simulink library "inp"  (R2021b)
settings: Solver=VariableStepAuto  StartTime=0.0  StopTime=10.0  RelTol=1e-3
undefined symbols (not defined in the file): C_TASK_5MS_S, FALSE, KINP_AcoreReadyToSlp_flg_ovrdflg, KINP_AcoreReadyToSlp_flg_ovrdval, KINP_AllowMovThd_OTA_enum_ovrdflg, KINP_AllowMovThd_OTA_enum_ovrdval, KINP_APSAngleTarget_Deg_ovrdflg, KINP_APSAngleTarget_Deg_ovrdval, KINP_APSDecReq_mps2_ovrdflg, KINP_APSDecReq_mps2_ovrdval, KINP_APSDecReqA_flg_ovrdflg, KINP_APSDecReqA_flg_ovrdval, KINP_APSDFLL_cm_ovrdflg, KINP_APSDFLL_cm_ovrdval, KINP_APSDFLR_cm_ovrdflg, KINP_APSDFLR_cm_ovrdval, KINP_APSDRLL_cm_ovrdflg, KINP_APSDRLL_cm_ovrdval, KINP_APSDRLR_cm_ovrdflg, KINP_APSDRLR_cm_ovrdval, KINP_APSExitCondition_enum_ovrdflg, KINP_APSExitCondition_enum_ovrdval, KINP_APSHWVer_enum_ovrdflg, KINP_APSHWVer_enum_ovrdval, KINP_APSProgressPCT_pct_ovrdflg, KINP_APSProgressPCT_pct_ovrdval, KINP_APSReq_enum_ovrdflg, KINP_APSReq_enum_ovrdval, KINP_APSRQDisplay_enum_ovrdflg, KINP_APSRQDisplay_enum_ovrdval, KINP_APSRqEPASCtrl_flg_ovrdflg, KINP_APSRqEPASCtrl_flg_ovrdval, KINP_APSShiftPosnReq_enum_ovrdval, KINP_APSShiftPosnReq_enum_ovrflg, KINP_APSSpeedCMD_kph_ovrdval, KINP_APSSpeedCMD_kph_ovrflg, KINP_APSStaSystem_enum_ovrdflg, KINP_APSStaSystem_enum_ovrdval, KINP_APSSWVer_enum_ovrdflg, KINP_APSSWVer_enum_ovrdval, KINP_APSVMCReqA_flg_ovrdval, KINP_APSVMCReqA_flg_ovrflg, KINP_APSVRqEPASCtrl_flg_ovrdflg, KINP_APSVRqEPASCtrl_flg_ovrdval, KINP_AuxBattVolmV_mV_ovrdflg, KINP_AuxBattVolmV_mV_ovrdval, KINP_CAASSta_enum_ovrdflg, KINP_CAASSta_enum_ovrdval, KINP_CAASVMCReqA_flg_ovrdval, KINP_CAASVMCReqA_flg_ovrflg, KINP_Chime_enum_ovrdflg, KINP_Chime_enum_ovrdval, KINP_ClearDTCcmd_flg_ovrdflg, KINP_ClearDTCcmd_flg_ovrdval, KINP_EvccAplusPwrUpReq_flg_ovrdflg, KINP_EvccAplusPwrUpReq_flg_ovrdval, KINP_LFID_raw_ovrdval, KINP_LFID_raw_ovrflg, KINP_LRID_raw_ovrdval, KINP_MemOffsetAccX_raw16_ovrdflg ... (+118)
libraries: FVT_lib x595, hcu_lib x1
(part 13 of 27)

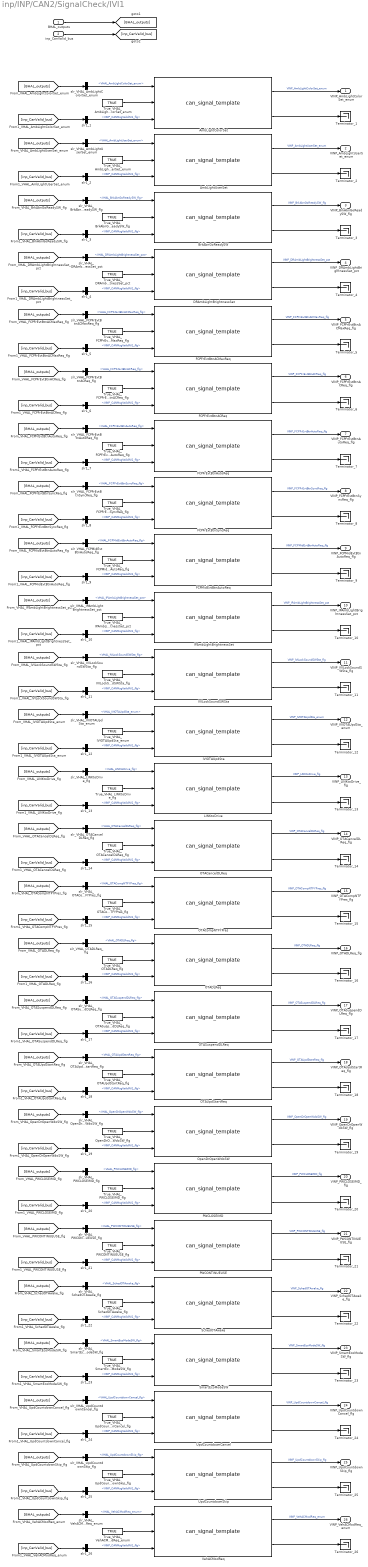
== system inp/INP/CAN2/SignalCheck/IVI1 ==
  BHAL_outputs : Inport
  inp_CanValid_bus : Inport  Port=2
  AmbLightColorSet : FVT_lib/inp/can_signal_template  SystemSampleTime=-1  VariantActivationTime=update diagram  Latency=0  AutoFrameSizeCalculation=off
      link override defval: Value=KINP_AmbLightColorSet_enum_defval
      link override fftdec: Value=KINP_AmbLightColorSet_enum_fftdec
      link override fftinc: Value=KINP_AmbLightColorSet_enum_fftinc
      link override fftlim: Value=KINP_AmbLightColorSet_enum_fftlim
      link override invalid: Value=KINP_AmbLightColorSet_enum_invalid
      link override ovrdflg: Value=KINP_AmbLightColorSet_enum_ovrdflg
      link override ovrdval: Value=KINP_AmbLightColorSet_enum_ovrdval
      link override setvalid: Value=KINP_AmbLightColorSet_enum_setvalid
      link override srvcflg: Value=KINP_AmbLightColorSet_enum_srvcflg
      link override srvcval: Value=KINP_AmbLightColorSet_enum_srvcval
  AmbLightUserSet : FVT_lib/inp/can_signal_template  SystemSampleTime=-1  VariantActivationTime=update diagram  Latency=0  AutoFrameSizeCalculation=off
      link override defval: Value=KINP_AmbLightUserSet_enum_defval
      link override fftdec: Value=KINP_AmbLightUserSet_enum_fftdec
      link override fftinc: Value=KINP_AmbLightUserSet_enum_fftinc
      link override fftlim: Value=KINP_AmbLightUserSet_enum_fftlim
      link override invalid: Value=KINP_AmbLightUserSet_enum_invalid
      link override ovrdflg: Value=KINP_AmbLightUserSet_enum_ovrdflg
      link override ovrdval: Value=KINP_AmbLightUserSet_enum_ovrdval
      link override setvalid: Value=KINP_AmbLightUserSet_enum_setvalid
      link override srvcflg: Value=KINP_AmbLightUserSet_enum_srvcflg
      link override srvcval: Value=KINP_AmbLightUserSet_enum_srvcval
  BrkAbnGoReadySW : FVT_lib/inp/can_signal_template  SystemSampleTime=-1  VariantActivationTime=update diagram  Latency=0  AutoFrameSizeCalculation=off
      link override defval: Value=KINP_BrkAbnGoReadySW_flg_defval
      link override fftdec: Value=KINP_BrkAbnGoReadySW_flg_fftdec
      link override fftinc: Value=KINP_BrkAbnGoReadySW_flg_fftinc
      link override fftlim: Value=KINP_BrkAbnGoReadySW_flg_fftlim
      link override invalid: Value=KINP_BrkAbnGoReadySW_flg_invalid
      link override ovrdflg: Value=KINP_BrkAbnGoReadySW_flg_ovrdflg
      link override ovrdval: Value=KINP_BrkAbnGoReadySW_flg_ovrdval
      link override setvalid: Value=KINP_BrkAbnGoReadySW_flg_setvalid
      link override srvcflg: Value=KINP_BrkAbnGoReadySW_flg_srvcflg
      link override srvcval: Value=KINP_BrkAbnGoReadySW_flg_srvcval
  DRAmbLightBrightnessSet : FVT_lib/inp/can_signal_template  SystemSampleTime=-1  VariantActivationTime=update diagram  Latency=0  AutoFrameSizeCalculation=off
      link override defval: Value=KINP_DRAmbLightBrightnessSet_pct_defval
      link override fftdec: Value=KINP_DRAmbLightBrightnessSet_pct_fftdec
      link override fftinc: Value=KINP_DRAmbLightBrightnessSet_pct_fftinc
      link override fftlim: Value=KINP_DRAmbLightBrightnessSet_pct_fftlim
      link override invalid: Value=KINP_DRAmbLightBrightnessSet_pct_invalid
      link override ovrdflg: Value=KINP_DRAmbLightBrightnessSet_pct_ovrdflg
      link override ovrdval: Value=KINP_DRAmbLightBrightnessSet_pct_ovrdval
      link override setvalid: Value=KINP_DRAmbLightBrightnessSet_pct_setvalid
      link override srvcflg: Value=KINP_DRAmbLightBrightnessSet_pct_srvcflg
      link override srvcval: Value=KINP_DRAmbLightBrightnessSet_pct_srvcval
  FCPFrEvtBtnACMaxReq : FVT_lib/inp/can_signal_template  SystemSampleTime=-1  VariantActivationTime=update diagram  Latency=0  AutoFrameSizeCalculation=off
      link override defval: Value=KINP_FCPFrEvtBtnACMaxReq_flg_defval
      link override fftdec: Value=KINP_FCPFrEvtBtnACMaxReq_flg_fftdec
      link override fftinc: Value=KINP_FCPFrEvtBtnACMaxReq_flg_fftinc
      link override fftlim: Value=KINP_FCPFrEvtBtnACMaxReq_flg_fftlim
      link override invalid: Value=KINP_FCPFrEvtBtnACMaxReq_flg_invalid
      link override ovrdflg: Value=KINP_FCPFrEvtBtnACMaxReq_flg_ovrdflg
      link override ovrdval: Value=KINP_FCPFrEvtBtnACMaxReq_flg_ovrdval
      link override setvalid: Value=KINP_FCPFrEvtBtnACMaxReq_flg_setvalid
      link override srvcflg: Value=KINP_FCPFrEvtBtnACMaxReq_flg_srvcflg
      link override srvcval: Value=KINP_FCPFrEvtBtnACMaxReq_flg_srvcval
  FCPFrEvtBtnACReq : FVT_lib/inp/can_signal_template  SystemSampleTime=-1  VariantActivationTime=update diagram  Latency=0  AutoFrameSizeCalculation=off
      link override defval: Value=KINP_FCPFrEvtBtnACReq_flg_defval
      link override fftdec: Value=KINP_FCPFrEvtBtnACReq_flg_fftdec
      link override fftinc: Value=KINP_FCPFrEvtBtnACReq_flg_fftinc
      link override fftlim: Value=KINP_FCPFrEvtBtnACReq_flg_fftlim
      link override invalid: Value=KINP_FCPFrEvtBtnACReq_flg_invalid
      link override ovrdflg: Value=KINP_FCPFrEvtBtnACReq_flg_ovrdflg
      link override ovrdval: Value=KINP_FCPFrEvtBtnACReq_flg_ovrdval
      link override setvalid: Value=KINP_FCPFrEvtBtnACReq_flg_setvalid
      link override srvcflg: Value=KINP_FCPFrEvtBtnACReq_flg_srvcflg
      link override srvcval: Value=KINP_FCPFrEvtBtnACReq_flg_srvcval
  FCPFrEvtBtnAutoReq : FVT_lib/inp/can_signal_template  SystemSampleTime=-1  VariantActivationTime=update diagram  Latency=0  AutoFrameSizeCalculation=off
      link override defval: Value=KINP_FCPFrEvtBtnAutoReq_flg_defval
      link override fftdec: Value=KINP_FCPFrEvtBtnAutoReq_flg_fftdec
      link override fftinc: Value=KINP_FCPFrEvtBtnAutoReq_flg_fftinc
      link override fftlim: Value=KINP_FCPFrEvtBtnAutoReq_flg_fftlim
      link override invalid: Value=KINP_FCPFrEvtBtnAutoReq_flg_invalid
      link override ovrdflg: Value=KINP_FCPFrEvtBtnAutoReq_flg_ovrdflg
      link override ovrdval: Value=KINP_FCPFrEvtBtnAutoReq_flg_ovrdval
      link override setvalid: Value=KINP_FCPFrEvtBtnAutoReq_flg_setvalid
      link override srvcflg: Value=KINP_FCPFrEvtBtnAutoReq_flg_srvcflg
      link override srvcval: Value=KINP_FCPFrEvtBtnAutoReq_flg_srvcval
  FCPFrEvtBtnSyncReq : FVT_lib/inp/can_signal_template  SystemSampleTime=-1  VariantActivationTime=update diagram  Latency=0  AutoFrameSizeCalculation=off
      link override defval: Value=KINP_FCPFrEvtBtnSyncReq_flg_defval
      link override fftdec: Value=KINP_FCPFrEvtBtnSyncReq_flg_fftdec
      link override fftinc: Value=KINP_FCPFrEvtBtnSyncReq_flg_fftinc
      link override fftlim: Value=KINP_FCPFrEvtBtnSyncReq_flg_fftlim
      link override invalid: Value=KINP_FCPFrEvtBtnSyncReq_flg_invalid
      link override ovrdflg: Value=KINP_FCPFrEvtBtnSyncReq_flg_ovrdflg
      link override ovrdval: Value=KINP_FCPFrEvtBtnSyncReq_flg_ovrdval
      link override setvalid: Value=KINP_FCPFrEvtBtnSyncReq_flg_setvalid
      link override srvcflg: Value=KINP_FCPFrEvtBtnSyncReq_flg_srvcflg
      link override srvcval: Value=KINP_FCPFrEvtBtnSyncReq_flg_srvcval
  FCPMidEvtBtnAutoReq : FVT_lib/inp/can_signal_template  SystemSampleTime=-1  VariantActivationTime=update diagram  Latency=0  AutoFrameSizeCalculation=off
      link override defval: Value=KINP_FCPMidEvtBtnAutoReq_flg_defval
      link override fftdec: Value=KINP_FCPMidEvtBtnAutoReq_flg_fftdec
      link override fftinc: Value=KINP_FCPMidEvtBtnAutoReq_flg_fftinc
      link override fftlim: Value=KINP_FCPMidEvtBtnAutoReq_flg_fftlim
      link override invalid: Value=KINP_FCPMidEvtBtnAutoReq_flg_invalid
      link override ovrdflg: Value=KINP_FCPMidEvtBtnAutoReq_flg_ovrdflg
      link override ovrdval: Value=KINP_FCPMidEvtBtnAutoReq_flg_ovrdval
      link override setvalid: Value=KINP_FCPMidEvtBtnAutoReq_flg_setvalid
      link override srvcflg: Value=KINP_FCPMidEvtBtnAutoReq_flg_srvcflg
      link override srvcval: Value=KINP_FCPMidEvtBtnAutoReq_flg_srvcval
  IPAmbLightBrightnessSet : FVT_lib/inp/can_signal_template  SystemSampleTime=-1  VariantActivationTime=update diagram  Latency=0  AutoFrameSizeCalculation=off
      link override defval: Value=KINP_IPAmbLightBrightnessSet_pct_defval
      link override fftdec: Value=KINP_IPAmbLightBrightnessSet_pct_fftdec
      link override fftinc: Value=KINP_IPAmbLightBrightnessSet_pct_fftinc
      link override fftlim: Value=KINP_IPAmbLightBrightnessSet_pct_fftlim
      link override invalid: Value=KINP_IPAmbLightBrightnessSet_pct_invalid
      link override ovrdflg: Value=KINP_IPAmbLightBrightnessSet_pct_ovrdflg
      link override ovrdval: Value=KINP_IPAmbLightBrightnessSet_pct_ovrdval
      link override setvalid: Value=KINP_IPAmbLightBrightnessSet_pct_setvalid
      link override srvcflg: Value=KINP_IPAmbLightBrightnessSet_pct_srvcflg
      link override srvcval: Value=KINP_IPAmbLightBrightnessSet_pct_srvcval
  IVILockSoundSWSta : FVT_lib/inp/can_signal_template  SystemSampleTime=-1  VariantActivationTime=update diagram  Latency=0  AutoFrameSizeCalculation=off
      link override defval: Value=KINP_IVILockSoundSWSta_flg_defval
      link override fftdec: Value=KINP_IVILockSoundSWSta_flg_fftdec
      link override fftinc: Value=KINP_IVILockSoundSWSta_flg_fftinc
      link override fftlim: Value=KINP_IVILockSoundSWSta_flg_fftlim
      link override invalid: Value=KINP_IVILockSoundSWSta_flg_invalid
      link override ovrdflg: Value=KINP_IVILockSoundSWSta_flg_ovrdflg
      link override ovrdval: Value=KINP_IVILockSoundSWSta_flg_ovrdval
      link override setvalid: Value=KINP_IVILockSoundSWSta_flg_setvalid
      link override srvcflg: Value=KINP_IVILockSoundSWSta_flg_srvcflg
      link override srvcval: Value=KINP_IVILockSoundSWSta_flg_srvcval
  IVIOTAUpdSta : FVT_lib/inp/can_signal_template  SystemSampleTime=-1  VariantActivationTime=update diagram  Latency=0  AutoFrameSizeCalculation=off
      link override defval: Value=KINP_IVIOTAUpdSta_enum_defval
      link override fftdec: Value=KINP_IVIOTAUpdSta_enum_fftdec
      link override fftinc: Value=KINP_IVIOTAUpdSta_enum_fftinc
      link override fftlim: Value=KINP_IVIOTAUpdSta_enum_fftlim
      link override invalid: Value=KINP_IVIOTAUpdSta_enum_invalid
      link override ovrdflg: Value=KINP_IVIOTAUpdSta_enum_ovrdflg
      link override ovrdval: Value=KINP_IVIOTAUpdSta_enum_ovrdval
      link override setvalid: Value=KINP_IVIOTAUpdSta_enum_setvalid
      link override srvcflg: Value=KINP_IVIOTAUpdSta_enum_srvcflg
      link override srvcval: Value=KINP_IVIOTAUpdSta_enum_srvcval
  LINKtoDrive : FVT_lib/inp/can_signal_template  SystemSampleTime=-1  VariantActivationTime=update diagram  Latency=0  AutoFrameSizeCalculation=off
      link override defval: Value=KINP_LINKtoDrive_flg_defval
      link override fftdec: Value=KINP_LINKtoDrive_flg_fftdec
      link override fftinc: Value=KINP_LINKtoDrive_flg_fftinc
      link override fftlim: Value=KINP_LINKtoDrive_flg_fftlim
      link override invalid: Value=KINP_LINKtoDrive_flg_invalid
      link override ovrdflg: Value=KINP_LINKtoDrive_flg_ovrdflg
      link override ovrdval: Value=KINP_LINKtoDrive_flg_ovrdval
      link override setvalid: Value=KINP_LINKtoDrive_flg_setvalid
      link override srvcflg: Value=KINP_LINKtoDrive_flg_srvcflg
      link override srvcval: Value=KINP_LINKtoDrive_flg_srvcval
  OTACancelDLReq : FVT_lib/inp/can_signal_template  SystemSampleTime=-1  VariantActivationTime=update diagram  Latency=0  AutoFrameSizeCalculation=off
      link override defval: Value=KINP_OTACancelDLReq_flg_defval
      link override fftdec: Value=KINP_OTACancelDLReq_flg_fftdec
      link override fftinc: Value=KINP_OTACancelDLReq_flg_fftinc
      link override fftlim: Value=KINP_OTACancelDLReq_flg_fftlim
      link override invalid: Value=KINP_OTACancelDLReq_flg_invalid
      link override ovrdflg: Value=KINP_OTACancelDLReq_flg_ovrdflg
      link override ovrdval: Value=KINP_OTACancelDLReq_flg_ovrdval
      link override setvalid: Value=KINP_OTACancelDLReq_flg_setvalid
      link override srvcflg: Value=KINP_OTACancelDLReq_flg_srvcflg
      link override srvcval: Value=KINP_OTACancelDLReq_flg_srvcval
  OTACompNTFYPres : FVT_lib/inp/can_signal_template  SystemSampleTime=-1  VariantActivationTime=update diagram  Latency=0  AutoFrameSizeCalculation=off
      link override defval: Value=KINP_OTACompNTFYPres_flg_defval
      link override fftdec: Value=KINP_OTACompNTFYPres_flg_fftdec
      link override fftinc: Value=KINP_OTACompNTFYPres_flg_fftinc
      link override fftlim: Value=KINP_OTACompNTFYPres_flg_fftlim
      link override invalid: Value=KINP_OTACompNTFYPres_flg_invalid
      link override ovrdflg: Value=KINP_OTACompNTFYPres_flg_ovrdflg
      link override ovrdval: Value=KINP_OTACompNTFYPres_flg_ovrdval
      link override setvalid: Value=KINP_OTACompNTFYPres_flg_setvalid
      link override srvcflg: Value=KINP_OTACompNTFYPres_flg_srvcflg
      link override srvcval: Value=KINP_OTACompNTFYPres_flg_srvcval
  OTADLReq : FVT_lib/inp/can_signal_template  SystemSampleTime=-1  VariantActivationTime=update diagram  Latency=0  AutoFrameSizeCalculation=off
      link override defval: Value=KINP_OTADLReq_flg_defval
      link override fftdec: Value=KINP_OTADLReq_flg_fftdec
      link override fftinc: Value=KINP_OTADLReq_flg_fftinc
      link override fftlim: Value=KINP_OTADLReq_flg_fftlim
      link override invalid: Value=KINP_OTADLReq_flg_invalid
      link override ovrdflg: Value=KINP_OTADLReq_flg_ovrdflg
      link override ovrdval: Value=KINP_OTADLReq_flg_ovrdval
      link override setvalid: Value=KINP_OTADLReq_flg_setvalid
      link override srvcflg: Value=KINP_OTADLReq_flg_srvcflg
      link override srvcval: Value=KINP_OTADLReq_flg_srvcval
  OTASuspendDLReq : FVT_lib/inp/can_signal_template  SystemSampleTime=-1  VariantActivationTime=update diagram  Latency=0  AutoFrameSizeCalculation=off
      link override defval: Value=KINP_OTASuspendDLReq_flg_defval
      link override fftdec: Value=KINP_OTASuspendDLReq_flg_fftdec
      link override fftinc: Value=KINP_OTASuspendDLReq_flg_fftinc
      link override fftlim: Value=KINP_OTASuspendDLReq_flg_fftlim
      link override invalid: Value=KINP_OTASuspendDLReq_flg_invalid
      link override ovrdflg: Value=KINP_OTASuspendDLReq_flg_ovrdflg
      link override ovrdval: Value=KINP_OTASuspendDLReq_flg_ovrdval
      link override setvalid: Value=KINP_OTASuspendDLReq_flg_setvalid
      link override srvcflg: Value=KINP_OTASuspendDLReq_flg_srvcflg
      link override srvcval: Value=KINP_OTASuspendDLReq_flg_srvcval
  OTAUpdStartReq : FVT_lib/inp/can_signal_template  SystemSampleTime=-1  VariantActivationTime=update diagram  Latency=0  AutoFrameSizeCalculation=off
      link override defval: Value=KINP_OTAUpdStartReq_flg_defval
      link override fftdec: Value=KINP_OTAUpdStartReq_flg_fftdec
      link override fftinc: Value=KINP_OTAUpdStartReq_flg_fftinc
      link override fftlim: Value=KINP_OTAUpdStartReq_flg_fftlim
      link override invalid: Value=KINP_OTAUpdStartReq_flg_invalid
      link override ovrdflg: Value=KINP_OTAUpdStartReq_flg_ovrdflg
      link override ovrdval: Value=KINP_OTAUpdStartReq_flg_ovrdval
      link override setvalid: Value=KINP_OTAUpdStartReq_flg_setvalid
      link override srvcflg: Value=KINP_OTAUpdStartReq_flg_srvcflg
      link override srvcval: Value=KINP_OTAUpdStartReq_flg_srvcval
  OpenDrOpenWdoSW : FVT_lib/inp/can_signal_template  SystemSampleTime=-1  VariantActivationTime=update diagram  Latency=0  AutoFrameSizeCalculation=off
      link override defval: Value=KINP_OpenDrOpenWdoSW_flg_defval
      link override fftdec: Value=KINP_OpenDrOpenWdoSW_flg_fftdec
      link override fftinc: Value=KINP_OpenDrOpenWdoSW_flg_fftinc
      link override fftlim: Value=KINP_OpenDrOpenWdoSW_flg_fftlim
      link override invalid: Value=KINP_OpenDrOpenWdoSW_flg_invalid
      link override ovrdflg: Value=KINP_OpenDrOpenWdoSW_flg_ovrdflg
      link override ovrdval: Value=KINP_OpenDrOpenWdoSW_flg_ovrdval
      link override setvalid: Value=KINP_OpenDrOpenWdoSW_flg_setvalid
      link override srvcflg: Value=KINP_OpenDrOpenWdoSW_flg_srvcflg
      link override srvcval: Value=KINP_OpenDrOpenWdoSW_flg_srvcval
  PWCLOSEIMD : FVT_lib/inp/can_signal_template  SystemSampleTime=-1  VariantActivationTime=update diagram  Latency=0  AutoFrameSizeCalculation=off
      link override defval: Value=KINP_PWCLOSEIMD_flg_defval
      link override fftdec: Value=KINP_PWCLOSEIMD_flg_fftdec
      link override fftinc: Value=KINP_PWCLOSEIMD_flg_fftinc
      link override fftlim: Value=KINP_PWCLOSEIMD_flg_fftlim
      link override invalid: Value=KINP_PWCLOSEIMD_flg_invalid
      link override ovrdflg: Value=KINP_PWCLOSEIMD_flg_ovrdflg
      link override ovrdval: Value=KINP_PWCLOSEIMD_flg_ovrdval
      link override setvalid: Value=KINP_PWCLOSEIMD_flg_setvalid
      link override srvcflg: Value=KINP_PWCLOSEIMD_flg_srvcflg
      link override srvcval: Value=KINP_PWCLOSEIMD_flg_srvcval
  PWCONTINUEUSE : FVT_lib/inp/can_signal_template  SystemSampleTime=-1  VariantActivationTime=update diagram  Latency=0  AutoFrameSizeCalculation=off
      link override defval: Value=KINP_PWCONTINUEUSE_flg_defval
      link override fftdec: Value=KINP_PWCONTINUEUSE_flg_fftdec
      link override fftinc: Value=KINP_PWCONTINUEUSE_flg_fftinc
      link override fftlim: Value=KINP_PWCONTINUEUSE_flg_fftlim
      link override invalid: Value=KINP_PWCONTINUEUSE_flg_invalid
      link override ovrdflg: Value=KINP_PWCONTINUEUSE_flg_ovrdflg
      link override ovrdval: Value=KINP_PWCONTINUEUSE_flg_ovrdval
      link override setvalid: Value=KINP_PWCONTINUEUSE_flg_setvalid
      link override srvcflg: Value=KINP_PWCONTINUEUSE_flg_srvcflg
      link override srvcval: Value=KINP_PWCONTINUEUSE_flg_srvcval
  SchedOTAwake : FVT_lib/inp/can_signal_template  SystemSampleTime=-1  VariantActivationTime=update diagram  Latency=0  AutoFrameSizeCalculation=off
      link override defval: Value=KINP_SchedOTAwake_flg_defval
      link override fftdec: Value=KINP_SchedOTAwake_flg_fftdec
      link override fftinc: Value=KINP_SchedOTAwake_flg_fftinc
      link override fftlim: Value=KINP_SchedOTAwake_flg_fftlim
      link override invalid: Value=KINP_SchedOTAwake_flg_invalid
      link override ovrdflg: Value=KINP_SchedOTAwake_flg_ovrdflg
      link override ovrdval: Value=KINP_SchedOTAwake_flg_ovrdval
      link override setvalid: Value=KINP_SchedOTAwake_flg_setvalid
      link override srvcflg: Value=KINP_SchedOTAwake_flg_srvcflg
      link override srvcval: Value=KINP_SchedOTAwake_flg_srvcval
  SmartEcoModeSW : FVT_lib/inp/can_signal_template  SystemSampleTime=-1  VariantActivationTime=update diagram  Latency=0  AutoFrameSizeCalculation=off
      link override defval: Value=KINP_SmartEcoModeSW_flg_defval
      link override fftdec: Value=KINP_SmartEcoModeSW_flg_fftdec
      link override fftinc: Value=KINP_SmartEcoModeSW_flg_fftinc
      link override fftlim: Value=KINP_SmartEcoModeSW_flg_fftlim
      link override invalid: Value=KINP_SmartEcoModeSW_flg_invalid
      link override ovrdflg: Value=KINP_SmartEcoModeSW_flg_ovrdflg
      link override ovrdval: Value=KINP_SmartEcoModeSW_flg_ovrdval
      link override setvalid: Value=KINP_SmartEcoModeSW_flg_setvalid
      link override srvcflg: Value=KINP_SmartEcoModeSW_flg_srvcflg
      link override srvcval: Value=KINP_SmartEcoModeSW_flg_srvcval
  Terminator_{1..26} (26 alike) : Terminator
  True_VHAL_AmbLightColorSet_enum : Constant  Value=TRUE  OutDataTypeStr=boolean
  True_VHAL_AmbLightUserSet_enum : Constant  Value=TRUE  OutDataTypeStr=boolean
  True_VHAL_BrkAbnGoReadySW_flg : Constant  Value=TRUE  OutDataTypeStr=boolean
  True_VHAL_DRAmbLightBrightnessSet_pct : Constant  Value=TRUE  OutDataTypeStr=boolean
  True_VHAL_FCPFrEvtBtnACMaxReq_flg : Constant  Value=TRUE  OutDataTypeStr=boolean
  True_VHAL_FCPFrEvtBtnACReq_flg : Constant  Value=TRUE  OutDataTypeStr=boolean
  True_VHAL_FCPFrEvtBtnAutoReq_flg : Constant  Value=TRUE  OutDataTypeStr=boolean
  True_VHAL_FCPFrEvtBtnSyncReq_flg : Constant  Value=TRUE  OutDataTypeStr=boolean
  True_VHAL_FCPMidEvtBtnAutoReq_flg : Constant  Value=TRUE  OutDataTypeStr=boolean
  True_VHAL_IPAmbLightBrightnessSet_pct : Constant  Value=TRUE  OutDataTypeStr=boolean
  True_VHAL_IVILockSoundSWSta_flg : Constant  Value=TRUE  OutDataTypeStr=boolean
  True_VHAL_IVIOTAUpdSta_enum : Constant  Value=TRUE  OutDataTypeStr=boolean
  True_VHAL_LINKtoDrive_flg : Constant  Value=TRUE  OutDataTypeStr=boolean
  True_VHAL_OTACancelDLReq_flg : Constant  Value=TRUE  OutDataTypeStr=boolean
  True_VHAL_OTACompNTFYPres_flg : Constant  Value=TRUE  OutDataTypeStr=boolean
  True_VHAL_OTADLReq_flg : Constant  Value=TRUE  OutDataTypeStr=boolean
  True_VHAL_OTASuspendDLReq_flg : Constant  Value=TRUE  OutDataTypeStr=boolean
  True_VHAL_OTAUpdStartReq_flg : Constant  Value=TRUE  OutDataTypeStr=boolean
  True_VHAL_OpenDrOpenWdoSW_flg : Constant  Value=TRUE  OutDataTypeStr=boolean
  True_VHAL_PWCLOSEIMD_flg : Constant  Value=TRUE  OutDataTypeStr=boolean
  True_VHAL_PWCONTINUEUSE_flg : Constant  Value=TRUE  OutDataTypeStr=boolean
  True_VHAL_SchedOTAwake_flg : Constant  Value=TRUE  OutDataTypeStr=boolean
  True_VHAL_SmartEcoModeSW_flg : Constant  Value=TRUE  OutDataTypeStr=boolean
  True_VHAL_UpdCountdownCancel_flg : Constant  Value=TRUE  OutDataTypeStr=boolean
  True_VHAL_UpdCountdownSkip_flg : Constant  Value=TRUE  OutDataTypeStr=boolean
  True_VHAL_VehACModReq_enum : Constant  Value=TRUE  OutDataTypeStr=boolean
  UpdCountdownCancel : FVT_lib/inp/can_signal_template  SystemSampleTime=-1  VariantActivationTime=update diagram  Latency=0  AutoFrameSizeCalculation=off
      link override defval: Value=KINP_UpdCountdownCancel_flg_defval
      link override fftdec: Value=KINP_UpdCountdownCancel_flg_fftdec
      link override fftinc: Value=KINP_UpdCountdownCancel_flg_fftinc
      link override fftlim: Value=KINP_UpdCountdownCancel_flg_fftlim
      link override invalid: Value=KINP_UpdCountdownCancel_flg_invalid
      link override ovrdflg: Value=KINP_UpdCountdownCancel_flg_ovrdflg
      link override ovrdval: Value=KINP_UpdCountdownCancel_flg_ovrdval
      link override setvalid: Value=KINP_UpdCountdownCancel_flg_setvalid
      link override srvcflg: Value=KINP_UpdCountdownCancel_flg_srvcflg
      link override srvcval: Value=KINP_UpdCountdownCancel_flg_srvcval
  UpdCountdownSkip : FVT_lib/inp/can_signal_template  SystemSampleTime=-1  VariantActivationTime=update diagram  Latency=0  AutoFrameSizeCalculation=off
      link override defval: Value=KINP_UpdCountdownSkip_flg_defval
      link override fftdec: Value=KINP_UpdCountdownSkip_flg_fftdec
      link override fftinc: Value=KINP_UpdCountdownSkip_flg_fftinc
      link override fftlim: Value=KINP_UpdCountdownSkip_flg_fftlim
      link override invalid: Value=KINP_UpdCountdownSkip_flg_invalid
      link override ovrdflg: Value=KINP_UpdCountdownSkip_flg_ovrdflg
      link override ovrdval: Value=KINP_UpdCountdownSkip_flg_ovrdval
      link override setvalid: Value=KINP_UpdCountdownSkip_flg_setvalid
      link override srvcflg: Value=KINP_UpdCountdownSkip_flg_srvcflg
      link override srvcval: Value=KINP_UpdCountdownSkip_flg_srvcval
  VehACModReq : FVT_lib/inp/can_signal_template  SystemSampleTime=-1  VariantActivationTime=update diagram  Latency=0  AutoFrameSizeCalculation=off
      link override defval: Value=KINP_VehACModReq_enum_defval
      link override fftdec: Value=KINP_VehACModReq_enum_fftdec
      link override fftinc: Value=KINP_VehACModReq_enum_fftinc
      link override fftlim: Value=KINP_VehACModReq_enum_fftlim
      link override invalid: Value=KINP_VehACModReq_enum_invalid
      link override ovrdflg: Value=KINP_VehACModReq_enum_ovrdflg
      link override ovrdval: Value=KINP_VehACModReq_enum_ovrdval
      link override setvalid: Value=KINP_VehACModReq_enum_setvalid
      link override srvcflg: Value=KINP_VehACModReq_enum_srvcflg
      link override srvcval: Value=KINP_VehACModReq_enum_srvcval
  slr1_{1..26} (26 alike) : BusSelector  OutputSignals=VINP_CANMsgValidIVI1_flg
  slr_VHAL_AmbLightColorSet_enum : BusSelector  OutputSignals=VHAL_AmbLightColorSet_enum
  slr_VHAL_AmbLightUserSet_enum : BusSelector  OutputSignals=VHAL_AmbLightUserSet_enum
  slr_VHAL_BrkAbnGoReadySW_flg : BusSelector  OutputSignals=VHAL_BrkAbnGoReadySW_flg
  slr_VHAL_DRAmbLightBrightnessSet_pct : BusSelector  OutputSignals=VHAL_DRAmbLightBrightnessSet_pct
  slr_VHAL_FCPFrEvtBtnACMaxReq_flg : BusSelector  OutputSignals=VHAL_FCPFrEvtBtnACMaxReq_flg
  slr_VHAL_FCPFrEvtBtnACReq_flg : BusSelector  OutputSignals=VHAL_FCPFrEvtBtnACReq_flg
  slr_VHAL_FCPFrEvtBtnAutoReq_flg : BusSelector  OutputSignals=VHAL_FCPFrEvtBtnAutoReq_flg
  slr_VHAL_FCPFrEvtBtnSyncReq_flg : BusSelector  OutputSignals=VHAL_FCPFrEvtBtnSyncReq_flg
  slr_VHAL_FCPMidEvtBtnAutoReq_flg : BusSelector  OutputSignals=VHAL_FCPMidEvtBtnAutoReq_flg
  slr_VHAL_IPAmbLightBrightnessSet_pct : BusSelector  OutputSignals=VHAL_IPAmbLightBrightnessSet_pct
  slr_VHAL_IVILockSoundSWSta_flg : BusSelector  OutputSignals=VHAL_IVILockSoundSWSta_flg
  slr_VHAL_IVIOTAUpdSta_enum : BusSelector  OutputSignals=VHAL_IVIOTAUpdSta_enum
  slr_VHAL_LINKtoDrive_flg : BusSelector  OutputSignals=VHAL_LINKtoDrive_flg
  slr_VHAL_OTACancelDLReq_flg : BusSelector  OutputSignals=VHAL_OTACancelDLReq_flg
  slr_VHAL_OTACompNTFYPres_flg : BusSelector  OutputSignals=VHAL_OTACompNTFYPres_flg
  slr_VHAL_OTADLReq_flg : BusSelector  OutputSignals=VHAL_OTADLReq_flg
  slr_VHAL_OTASuspendDLReq_flg : BusSelector  OutputSignals=VHAL_OTASuspendDLReq_flg
  slr_VHAL_OTAUpdStartReq_flg : BusSelector  OutputSignals=VHAL_OTAUpdStartReq_flg
  slr_VHAL_OpenDrOpenWdoSW_flg : BusSelector  OutputSignals=VHAL_OpenDrOpenWdoSW_flg
  slr_VHAL_PWCLOSEIMD_flg : BusSelector  OutputSignals=VHAL_PWCLOSEIMD_flg
  slr_VHAL_PWCONTINUEUSE_flg : BusSelector  OutputSignals=VHAL_PWCONTINUEUSE_flg
  slr_VHAL_SchedOTAwake_flg : BusSelector  OutputSignals=VHAL_SchedOTAwake_flg
  slr_VHAL_SmartEcoModeSW_flg : BusSelector  OutputSignals=VHAL_SmartEcoModeSW_flg
  slr_VHAL_UpdCountdownCancel_flg : BusSelector  OutputSignals=VHAL_UpdCountdownCancel_flg
  slr_VHAL_UpdCountdownSkip_flg : BusSelector  OutputSignals=VHAL_UpdCountdownSkip_flg
  slr_VHAL_VehACModReq_enum : BusSelector  OutputSignals=VHAL_VehACModReq_enum
  VINP_AmbLightColorSet_enum : Outport
  VINP_AmbLightUserSet_enum : Outport  Port=2
  VINP_BrkAbnGoReadySW_flg : Outport  Port=3
  VINP_DRAmbLightBrightnessSet_pct : Outport  Port=4
  VINP_FCPFrEvtBtnACMaxReq_flg : Outport  Port=5
  VINP_FCPFrEvtBtnACReq_flg : Outport  Port=6
  VINP_FCPFrEvtBtnAutoReq_flg : Outport  Port=7
  VINP_FCPFrEvtBtnSyncReq_flg : Outport  Port=8
  VINP_FCPMidEvtBtnAutoReq_flg : Outport  Port=9
  VINP_IPAmbLightBrightnessSet_pct : Outport  Port=10
  VINP_IVILockSoundSWSta_flg : Outport  Port=11
  VINP_IVIOTAUpdSta_enum : Outport  Port=12
  VINP_LINKtoDrive_flg : Outport  Port=13
  VINP_OTACancelDLReq_flg : Outport  Port=14
  VINP_OTACompNTFYPres_flg : Outport  Port=15
  VINP_OTADLReq_flg : Outport  Port=16
  VINP_OTASuspendDLReq_flg : Outport  Port=17
  VINP_OTAUpdStartReq_flg : Outport  Port=18
  VINP_OpenDrOpenWdoSW_flg : Outport  Port=19
  VINP_PWCLOSEIMD_flg : Outport  Port=20
  VINP_PWCONTINUEUSE_flg : Outport  Port=21
  VINP_SchedOTAwake_flg : Outport  Port=22
  VINP_SmartEcoModeSW_flg : Outport  Port=23
  VINP_UpdCountdownCancel_flg : Outport  Port=24
  VINP_UpdCountdownSkip_flg : Outport  Port=25
  VINP_VehACModReq_enum : Outport  Port=26
  wires:
  BHAL_outputs/1 -> [BHAL_outputs]
  inp_CanValid_bus/1 -> [inp_CanValid_bus]
  [BHAL_outputs] -> slr_VHAL_AmbLightColorSet_enum/1
  slr_VHAL_AmbLightColorSet_enum/1 -> AmbLightColorSet/1  "<VHAL_AmbLightColorSet_enum>"
  True_VHAL_AmbLightColorSet_enum/1 -> AmbLightColorSet/2
  [inp_CanValid_bus] -> slr1_1/1
  slr1_1/1 -> AmbLightColorSet/3  "<VINP_CANMsgValidIVI1_flg>"
  AmbLightColorSet/1 -> VINP_AmbLightColorSet_enum/1  "VINP_AmbLightColorSet_enum"
  AmbLightColorSet/2 -> Terminator_1/1
  [BHAL_outputs] -> slr_VHAL_AmbLightUserSet_enum/1
  slr_VHAL_AmbLightUserSet_enum/1 -> AmbLightUserSet/1  "<VHAL_AmbLightUserSet_enum>"
  True_VHAL_AmbLightUserSet_enum/1 -> AmbLightUserSet/2
  [inp_CanValid_bus] -> slr1_2/1
  slr1_2/1 -> AmbLightUserSet/3  "<VINP_CANMsgValidIVI1_flg>"
  AmbLightUserSet/1 -> VINP_AmbLightUserSet_enum/1  "VINP_AmbLightUserSet_enum"
  AmbLightUserSet/2 -> Terminator_2/1
  [BHAL_outputs] -> slr_VHAL_BrkAbnGoReadySW_flg/1
  slr_VHAL_BrkAbnGoReadySW_flg/1 -> BrkAbnGoReadySW/1  "<VHAL_BrkAbnGoReadySW_flg>"
  True_VHAL_BrkAbnGoReadySW_flg/1 -> BrkAbnGoReadySW/2
  [inp_CanValid_bus] -> slr1_3/1
  slr1_3/1 -> BrkAbnGoReadySW/3  "<VINP_CANMsgValidIVI1_flg>"
  BrkAbnGoReadySW/1 -> VINP_BrkAbnGoReadySW_flg/1  "VINP_BrkAbnGoReadySW_flg"
  BrkAbnGoReadySW/2 -> Terminator_3/1
  [BHAL_outputs] -> slr_VHAL_DRAmbLightBrightnessSet_pct/1
  slr_VHAL_DRAmbLightBrightnessSet_pct/1 -> DRAmbLightBrightnessSet/1  "<VHAL_DRAmbLightBrightnessSet_pct>"
  True_VHAL_DRAmbLightBrightnessSet_pct/1 -> DRAmbLightBrightnessSet/2
  [inp_CanValid_bus] -> slr1_4/1
  slr1_4/1 -> DRAmbLightBrightnessSet/3  "<VINP_CANMsgValidIVI1_flg>"
  DRAmbLightBrightnessSet/1 -> VINP_DRAmbLightBrightnessSet_pct/1  "VINP_DRAmbLightBrightnessSet_pct"
  DRAmbLightBrightnessSet/2 -> Terminator_4/1
  [BHAL_outputs] -> slr_VHAL_FCPFrEvtBtnACMaxReq_flg/1
  slr_VHAL_FCPFrEvtBtnACMaxReq_flg/1 -> FCPFrEvtBtnACMaxReq/1  "<VHAL_FCPFrEvtBtnACMaxReq_flg>"
  True_VHAL_FCPFrEvtBtnACMaxReq_flg/1 -> FCPFrEvtBtnACMaxReq/2
  [inp_CanValid_bus] -> slr1_5/1
  slr1_5/1 -> FCPFrEvtBtnACMaxReq/3  "<VINP_CANMsgValidIVI1_flg>"
  FCPFrEvtBtnACMaxReq/1 -> VINP_FCPFrEvtBtnACMaxReq_flg/1  "VINP_FCPFrEvtBtnACMaxReq_flg"
  FCPFrEvtBtnACMaxReq/2 -> Terminator_5/1
  [BHAL_outputs] -> slr_VHAL_FCPFrEvtBtnACReq_flg/1
  slr_VHAL_FCPFrEvtBtnACReq_flg/1 -> FCPFrEvtBtnACReq/1  "<VHAL_FCPFrEvtBtnACReq_flg>"
  True_VHAL_FCPFrEvtBtnACReq_flg/1 -> FCPFrEvtBtnACReq/2
  [inp_CanValid_bus] -> slr1_6/1
  slr1_6/1 -> FCPFrEvtBtnACReq/3  "<VINP_CANMsgValidIVI1_flg>"
  FCPFrEvtBtnACReq/1 -> VINP_FCPFrEvtBtnACReq_flg/1  "VINP_FCPFrEvtBtnACReq_flg"
  FCPFrEvtBtnACReq/2 -> Terminator_6/1
  [BHAL_outputs] -> slr_VHAL_FCPFrEvtBtnAutoReq_flg/1
  slr_VHAL_FCPFrEvtBtnAutoReq_flg/1 -> FCPFrEvtBtnAutoReq/1  "<VHAL_FCPFrEvtBtnAutoReq_flg>"
  True_VHAL_FCPFrEvtBtnAutoReq_flg/1 -> FCPFrEvtBtnAutoReq/2
  [inp_CanValid_bus] -> slr1_7/1
  slr1_7/1 -> FCPFrEvtBtnAutoReq/3  "<VINP_CANMsgValidIVI1_flg>"
  FCPFrEvtBtnAutoReq/1 -> VINP_FCPFrEvtBtnAutoReq_flg/1  "VINP_FCPFrEvtBtnAutoReq_flg"
  FCPFrEvtBtnAutoReq/2 -> Terminator_7/1
  [BHAL_outputs] -> slr_VHAL_FCPFrEvtBtnSyncReq_flg/1
  slr_VHAL_FCPFrEvtBtnSyncReq_flg/1 -> FCPFrEvtBtnSyncReq/1  "<VHAL_FCPFrEvtBtnSyncReq_flg>"
  True_VHAL_FCPFrEvtBtnSyncReq_flg/1 -> FCPFrEvtBtnSyncReq/2
  [inp_CanValid_bus] -> slr1_8/1
  slr1_8/1 -> FCPFrEvtBtnSyncReq/3  "<VINP_CANMsgValidIVI1_flg>"
  FCPFrEvtBtnSyncReq/1 -> VINP_FCPFrEvtBtnSyncReq_flg/1  "VINP_FCPFrEvtBtnSyncReq_flg"
  FCPFrEvtBtnSyncReq/2 -> Terminator_8/1
  [BHAL_outputs] -> slr_VHAL_FCPMidEvtBtnAutoReq_flg/1
  slr_VHAL_FCPMidEvtBtnAutoReq_flg/1 -> FCPMidEvtBtnAutoReq/1  "<VHAL_FCPMidEvtBtnAutoReq_flg>"
  True_VHAL_FCPMidEvtBtnAutoReq_flg/1 -> FCPMidEvtBtnAutoReq/2
  [inp_CanValid_bus] -> slr1_9/1
  slr1_9/1 -> FCPMidEvtBtnAutoReq/3  "<VINP_CANMsgValidIVI1_flg>"
  FCPMidEvtBtnAutoReq/1 -> VINP_FCPMidEvtBtnAutoReq_flg/1  "VINP_FCPMidEvtBtnAutoReq_flg"
  FCPMidEvtBtnAutoReq/2 -> Terminator_9/1
  [BHAL_outputs] -> slr_VHAL_IPAmbLightBrightnessSet_pct/1
  slr_VHAL_IPAmbLightBrightnessSet_pct/1 -> IPAmbLightBrightnessSet/1  "<VHAL_IPAmbLightBrightnessSet_pct>"
  True_VHAL_IPAmbLightBrightnessSet_pct/1 -> IPAmbLightBrightnessSet/2
  [inp_CanValid_bus] -> slr1_10/1
  slr1_10/1 -> IPAmbLightBrightnessSet/3  "<VINP_CANMsgValidIVI1_flg>"
  IPAmbLightBrightnessSet/1 -> VINP_IPAmbLightBrightnessSet_pct/1  "VINP_IPAmbLightBrightnessSet_pct"
  IPAmbLightBrightnessSet/2 -> Terminator_10/1
  [BHAL_outputs] -> slr_VHAL_IVILockSoundSWSta_flg/1
  slr_VHAL_IVILockSoundSWSta_flg/1 -> IVILockSoundSWSta/1  "<VHAL_IVILockSoundSWSta_flg>"
  True_VHAL_IVILockSoundSWSta_flg/1 -> IVILockSoundSWSta/2
  [inp_CanValid_bus] -> slr1_11/1
  slr1_11/1 -> IVILockSoundSWSta/3  "<VINP_CANMsgValidIVI1_flg>"
  IVILockSoundSWSta/1 -> VINP_IVILockSoundSWSta_flg/1  "VINP_IVILockSoundSWSta_flg"
  IVILockSoundSWSta/2 -> Terminator_11/1
  [BHAL_outputs] -> slr_VHAL_IVIOTAUpdSta_enum/1
  slr_VHAL_IVIOTAUpdSta_enum/1 -> IVIOTAUpdSta/1  "<VHAL_IVIOTAUpdSta_enum>"
  True_VHAL_IVIOTAUpdSta_enum/1 -> IVIOTAUpdSta/2
  [inp_CanValid_bus] -> slr1_12/1
  slr1_12/1 -> IVIOTAUpdSta/3  "<VINP_CANMsgValidIVI1_flg>"
  IVIOTAUpdSta/1 -> VINP_IVIOTAUpdSta_enum/1  "VINP_IVIOTAUpdSta_enum"
  IVIOTAUpdSta/2 -> Terminator_12/1
  [BHAL_outputs] -> slr_VHAL_LINKtoDrive_flg/1
  slr_VHAL_LINKtoDrive_flg/1 -> LINKtoDrive/1  "<VHAL_LINKtoDrive_flg>"
  True_VHAL_LINKtoDrive_flg/1 -> LINKtoDrive/2
  [inp_CanValid_bus] -> slr1_13/1
  slr1_13/1 -> LINKtoDrive/3  "<VINP_CANMsgValidIVI1_flg>"
  LINKtoDrive/1 -> VINP_LINKtoDrive_flg/1  "VINP_LINKtoDrive_flg"
  LINKtoDrive/2 -> Terminator_13/1
  [BHAL_outputs] -> slr_VHAL_OTACancelDLReq_flg/1
  slr_VHAL_OTACancelDLReq_flg/1 -> OTACancelDLReq/1  "<VHAL_OTACancelDLReq_flg>"
  True_VHAL_OTACancelDLReq_flg/1 -> OTACancelDLReq/2
  [inp_CanValid_bus] -> slr1_14/1
  slr1_14/1 -> OTACancelDLReq/3  "<VINP_CANMsgValidIVI1_flg>"
  OTACancelDLReq/1 -> VINP_OTACancelDLReq_flg/1  "VINP_OTACancelDLReq_flg"
  OTACancelDLReq/2 -> Terminator_14/1
  [BHAL_outputs] -> slr_VHAL_OTACompNTFYPres_flg/1
  slr_VHAL_OTACompNTFYPres_flg/1 -> OTACompNTFYPres/1  "<VHAL_OTACompNTFYPres_flg>"
  True_VHAL_OTACompNTFYPres_flg/1 -> OTACompNTFYPres/2
  [inp_CanValid_bus] -> slr1_15/1
  slr1_15/1 -> OTACompNTFYPres/3  "<VINP_CANMsgValidIVI1_flg>"
  OTACompNTFYPres/1 -> VINP_OTACompNTFYPres_flg/1  "VINP_OTACompNTFYPres_flg"
  OTACompNTFYPres/2 -> Terminator_15/1
  [BHAL_outputs] -> slr_VHAL_OTADLReq_flg/1
  slr_VHAL_OTADLReq_flg/1 -> OTADLReq/1  "<VHAL_OTADLReq_flg>"
  True_VHAL_OTADLReq_flg/1 -> OTADLReq/2
  [inp_CanValid_bus] -> slr1_16/1
  slr1_16/1 -> OTADLReq/3  "<VINP_CANMsgValidIVI1_flg>"
  OTADLReq/1 -> VINP_OTADLReq_flg/1  "VINP_OTADLReq_flg"
  OTADLReq/2 -> Terminator_16/1
  [BHAL_outputs] -> slr_VHAL_OTASuspendDLReq_flg/1
  slr_VHAL_OTASuspendDLReq_flg/1 -> OTASuspendDLReq/1  "<VHAL_OTASuspendDLReq_flg>"
  True_VHAL_OTASuspendDLReq_flg/1 -> OTASuspendDLReq/2
  [inp_CanValid_bus] -> slr1_17/1
  slr1_17/1 -> OTASuspendDLReq/3  "<VINP_CANMsgValidIVI1_flg>"
  OTASuspendDLReq/1 -> VINP_OTASuspendDLReq_flg/1  "VINP_OTASuspendDLReq_flg"
  OTASuspendDLReq/2 -> Terminator_17/1
  [BHAL_outputs] -> slr_VHAL_OTAUpdStartReq_flg/1
  slr_VHAL_OTAUpdStartReq_flg/1 -> OTAUpdStartReq/1  "<VHAL_OTAUpdStartReq_flg>"
  True_VHAL_OTAUpdStartReq_flg/1 -> OTAUpdStartReq/2
  [inp_CanValid_bus] -> slr1_18/1
  slr1_18/1 -> OTAUpdStartReq/3  "<VINP_CANMsgValidIVI1_flg>"
  OTAUpdStartReq/1 -> VINP_OTAUpdStartReq_flg/1  "VINP_OTAUpdStartReq_flg"
  OTAUpdStartReq/2 -> Terminator_18/1
  [BHAL_outputs] -> slr_VHAL_OpenDrOpenWdoSW_flg/1
  slr_VHAL_OpenDrOpenWdoSW_flg/1 -> OpenDrOpenWdoSW/1  "<VHAL_OpenDrOpenWdoSW_flg>"
  True_VHAL_OpenDrOpenWdoSW_flg/1 -> OpenDrOpenWdoSW/2
  [inp_CanValid_bus] -> slr1_19/1
  slr1_19/1 -> OpenDrOpenWdoSW/3  "<VINP_CANMsgValidIVI1_flg>"
  OpenDrOpenWdoSW/1 -> VINP_OpenDrOpenWdoSW_flg/1  "VINP_OpenDrOpenWdoSW_flg"
  OpenDrOpenWdoSW/2 -> Terminator_19/1
  [BHAL_outputs] -> slr_VHAL_PWCLOSEIMD_flg/1
  slr_VHAL_PWCLOSEIMD_flg/1 -> PWCLOSEIMD/1  "<VHAL_PWCLOSEIMD_flg>"
  True_VHAL_PWCLOSEIMD_flg/1 -> PWCLOSEIMD/2
  [inp_CanValid_bus] -> slr1_20/1
  slr1_20/1 -> PWCLOSEIMD/3  "<VINP_CANMsgValidIVI1_flg>"
  PWCLOSEIMD/1 -> VINP_PWCLOSEIMD_flg/1  "VINP_PWCLOSEIMD_flg"
  PWCLOSEIMD/2 -> Terminator_20/1
  [BHAL_outputs] -> slr_VHAL_PWCONTINUEUSE_flg/1
  slr_VHAL_PWCONTINUEUSE_flg/1 -> PWCONTINUEUSE/1  "<VHAL_PWCONTINUEUSE_flg>"
  True_VHAL_PWCONTINUEUSE_flg/1 -> PWCONTINUEUSE/2
  [inp_CanValid_bus] -> slr1_21/1
  slr1_21/1 -> PWCONTINUEUSE/3  "<VINP_CANMsgValidIVI1_flg>"
  PWCONTINUEUSE/1 -> VINP_PWCONTINUEUSE_flg/1  "VINP_PWCONTINUEUSE_flg"
  PWCONTINUEUSE/2 -> Terminator_21/1
  [BHAL_outputs] -> slr_VHAL_SchedOTAwake_flg/1
  slr_VHAL_SchedOTAwake_flg/1 -> SchedOTAwake/1  "<VHAL_SchedOTAwake_flg>"
  True_VHAL_SchedOTAwake_flg/1 -> SchedOTAwake/2
  [inp_CanValid_bus] -> slr1_22/1
  slr1_22/1 -> SchedOTAwake/3  "<VINP_CANMsgValidIVI1_flg>"
  SchedOTAwake/1 -> VINP_SchedOTAwake_flg/1  "VINP_SchedOTAwake_flg"
  SchedOTAwake/2 -> Terminator_22/1
  [BHAL_outputs] -> slr_VHAL_SmartEcoModeSW_flg/1
  slr_VHAL_SmartEcoModeSW_flg/1 -> SmartEcoModeSW/1  "<VHAL_SmartEcoModeSW_flg>"
  True_VHAL_SmartEcoModeSW_flg/1 -> SmartEcoModeSW/2
  [inp_CanValid_bus] -> slr1_23/1
  slr1_23/1 -> SmartEcoModeSW/3  "<VINP_CANMsgValidIVI1_flg>"
  SmartEcoModeSW/1 -> VINP_SmartEcoModeSW_flg/1  "VINP_SmartEcoModeSW_flg"
  SmartEcoModeSW/2 -> Terminator_23/1
  [BHAL_outputs] -> slr_VHAL_UpdCountdownCancel_flg/1
  slr_VHAL_UpdCountdownCancel_flg/1 -> UpdCountdownCancel/1  "<VHAL_UpdCountdownCancel_flg>"
  True_VHAL_UpdCountdownCancel_flg/1 -> UpdCountdownCancel/2
  [inp_CanValid_bus] -> slr1_24/1
  slr1_24/1 -> UpdCountdownCancel/3  "<VINP_CANMsgValidIVI1_flg>"
  UpdCountdownCancel/1 -> VINP_UpdCountdownCancel_flg/1  "VINP_UpdCountdownCancel_flg"
  UpdCountdownCancel/2 -> Terminator_24/1
  [BHAL_outputs] -> slr_VHAL_UpdCountdownSkip_flg/1
  slr_VHAL_UpdCountdownSkip_flg/1 -> UpdCountdownSkip/1  "<VHAL_UpdCountdownSkip_flg>"
  True_VHAL_UpdCountdownSkip_flg/1 -> UpdCountdownSkip/2
  [inp_CanValid_bus] -> slr1_25/1
  slr1_25/1 -> UpdCountdownSkip/3  "<VINP_CANMsgValidIVI1_flg>"
  UpdCountdownSkip/1 -> VINP_UpdCountdownSkip_flg/1  "VINP_UpdCountdownSkip_flg"
  UpdCountdownSkip/2 -> Terminator_25/1
  [BHAL_outputs] -> slr_VHAL_VehACModReq_enum/1
  slr_VHAL_VehACModReq_enum/1 -> VehACModReq/1  "<VHAL_VehACModReq_enum>"
  True_VHAL_VehACModReq_enum/1 -> VehACModReq/2
  [inp_CanValid_bus] -> slr1_26/1
  slr1_26/1 -> VehACModReq/3  "<VINP_CANMsgValidIVI1_flg>"
  VehACModReq/1 -> VINP_VehACModReq_enum/1  "VINP_VehACModReq_enum"
  VehACModReq/2 -> Terminator_26/1
